simulink library "libEngineAngMomSpecs"  (R2020b)
settings: Solver=VariableStepAuto  StartTime=0.0  StopTime=10.0  RelTol=1e-3
undefined symbols (not defined in the file): data
settings Model: Creator=caatay  LastModifiedBy=caatay

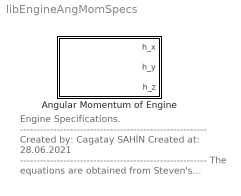
== system libEngineAngMomSpecs ==
  note: Engine Specifications.
      | --------------------------------------------------------
      | Created by: Cagatay SAHİN
      | Created at: 28.06.2021
      | --------------------------------------------------------
      | The equations are obtained from
      | Steven's textbook.
      | The reference book can be found in
      | "references folder".
      | --------------------------------------------------------
      | for question:
      | cagataysahin44@gmail.com
  Angular Momentum of Engine : Subsystem  mask(Engine Model - Angular Momentum of Engine){data=data}
      mask prompts: data "Angular Moment of Engine Data"
      mask help: Aircraft's engine specification in Imperical units
      mask Help:
      | This block is used for getting engine's angular momentum specifications.
      | --------------------------------------------------------------------------------------------------------------------------------------------------
      | Output of the function:
      | 	h_ii: Angular Momentum of Engine on X-Y-Z Axes
      | --------------------------------------------------------------------------------------------------------------------------------------------------
      | All equations can be found in Steven's text book. Reference can be found in "literature" subfolder.
      | for question: "cagataysahin44@gmail.com"
      mask Display:
      | port_label('output', 1, 'h_{x}', 'texmode', 'on');
      | port_label('output', 2, 'h_{y}', 'texmode', 'on');
      | port_label('output', 3, 'h_{z}', 'texmode', 'on');

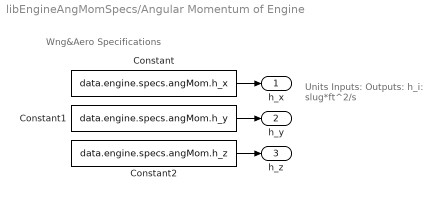
== system libEngineAngMomSpecs/Angular Momentum of Engine ==
  note: Units
      | Inputs:
      |
      | Outputs:
      | h_i: slug*ft^2/s
  note: Wng&Aero Specifications
  Constant : Constant  Value=data.engine.specs.angMom.h_x
  Constant1 : Constant  Value=data.engine.specs.angMom.h_y
  Constant2 : Constant  Value=data.engine.specs.angMom.h_z
  h_x : Outport  VectorParamsAs1DForOutWhenUnconnected=off
  h_y : Outport  Port=2  VectorParamsAs1DForOutWhenUnconnected=off
  h_z : Outport  Port=3  VectorParamsAs1DForOutWhenUnconnected=off
  wires:
  Constant/1 -> h_x/1
  Constant1/1 -> h_y/1
  Constant2/1 -> h_z/1
